simulink model "rx_channelizer_AIE"  (R2024a)
settings: Solver=VariableStepAuto  StartTime=0.0  StopTime=1280*12/fs  RelTol=1e-3
PreLoadFcn:
  | ch_rate = 41e6; % per channel sample rate
  | num_ch = 32;
  | 
  | % note:  6 coeffs/ch;
  | fs = ch_rate*num_ch;
  | sample_rate = 1/fs;
  | base_freq=1e6; % what base channel frequency to modulate?
  | 
  | generate_prototype_FIR; % create FIR coeffs
values from neighbouring files (symbols this model uses):
  ch0f = int16(scale*ch0)    [generate_prototype_FIR.m]
  ch10f = int16(scale*ch10)    [generate_prototype_FIR.m]
  ch11f = int16(scale*ch11)    [generate_prototype_FIR.m]
  ch12f = int16(scale*ch12)    [generate_prototype_FIR.m]
  ch13f = int16(scale*ch13)    [generate_prototype_FIR.m]
  ch14f = int16(scale*ch14)    [generate_prototype_FIR.m]
  ch15f = int16(scale*ch15)    [generate_prototype_FIR.m]
  ch16f = int16(scale*ch16)    [generate_prototype_FIR.m]
  ch17f = int16(scale*ch17)    [generate_prototype_FIR.m]
  ch18f = int16(scale*ch18)    [generate_prototype_FIR.m]
  ch19f = int16(scale*ch19)    [generate_prototype_FIR.m]
  ch1f = int16(scale*ch1)    [generate_prototype_FIR.m]
  ch20f = int16(scale*ch20)    [generate_prototype_FIR.m]
  ch21f = int16(scale*ch21)    [generate_prototype_FIR.m]
  ch22f = int16(scale*ch22)    [generate_prototype_FIR.m]
  ch23f = int16(scale*ch23)    [generate_prototype_FIR.m]
  ch24f = int16(scale*ch24)    [generate_prototype_FIR.m]
  ch25f = int16(scale*ch25)    [generate_prototype_FIR.m]
  ch26f = int16(scale*ch26)    [generate_prototype_FIR.m]
  ch27f = int16(scale*ch27)    [generate_prototype_FIR.m]
  ch28f = int16(scale*ch28)    [generate_prototype_FIR.m]
  ch29f = int16(scale*ch29)    [generate_prototype_FIR.m]
  ch2f = int16(scale*ch2)    [generate_prototype_FIR.m]
  ch30f = int16(scale*ch30)    [generate_prototype_FIR.m]
  ch31f = int16(scale*ch31)    [generate_prototype_FIR.m]
  ch3f = int16(scale*ch3)    [generate_prototype_FIR.m]
  ch4f = int16(scale*ch4)    [generate_prototype_FIR.m]
  ch5f = int16(scale*ch5)    [generate_prototype_FIR.m]
  ch6f = int16(scale*ch6)    [generate_prototype_FIR.m]
  ch7f = int16(scale*ch7)    [generate_prototype_FIR.m]
  ch8f = int16(scale*ch8)    [generate_prototype_FIR.m]
  ch9f = int16(scale*ch9)    [generate_prototype_FIR.m]
  filtAIE1_fp = filtAIE2_fp'    [generate_prototype_FIR.m]
undefined symbols (not defined in the file or in its folder): None, PLclk, S, vsva2197, xcvc1902
libraries: aieBasic x12, dspsrcs4 x4, aieUtilities x4, aieDSP x2, dspmlti4 x1, dspxfrm3 x1, vmcUtilities x1
settings Model: Creator=mmi  LastModifiedBy=robg
settings SolverCC: AlgebraicLoopSolver=TrustRegion
settings DebuggingCC: UnconnectedInputMsg=warning  UnconnectedOutputMsg=warning  UnconnectedLineMsg=warning
settings HardwareCC: ProdBitPerPointer=32  ProdBitPerSizeT=32  ProdBitPerPtrDiffT=32  ProdLargestAtomicFloat=None  ProdIntDivRoundTo=Undefined  ProdEndianess=Unspecified  ProdWordSize=32  ProdHWDeviceType=ASIC/FPGA->ASIC/FPGA  TargetBitPerLong=64  TargetBitPerPointer=64  TargetBitPerSizeT=64  TargetBitPerPtrDiffT=64  TargetLongLongMode=on  TargetIntDivRoundTo=Zero  TargetEndianess=LittleEndian  TargetWordSize=64  TargetHWDeviceType=Custom Processor->MATLAB Host Computer  ProdEqTarget=off
settings ModelReferenceCC: EnableRefExpFcnMdlSchedulingChecks=on
settings RTWCC: GPUComputeCapability=3.5  DLArmComputeVersion=19.05
settings ConfigComp: CovBoundaryAbsTol=1.0e-5

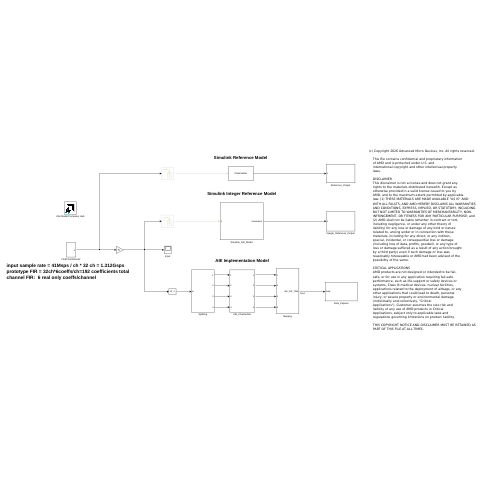
[thumbnail: Simulink's stored preview of the top-level diagram]
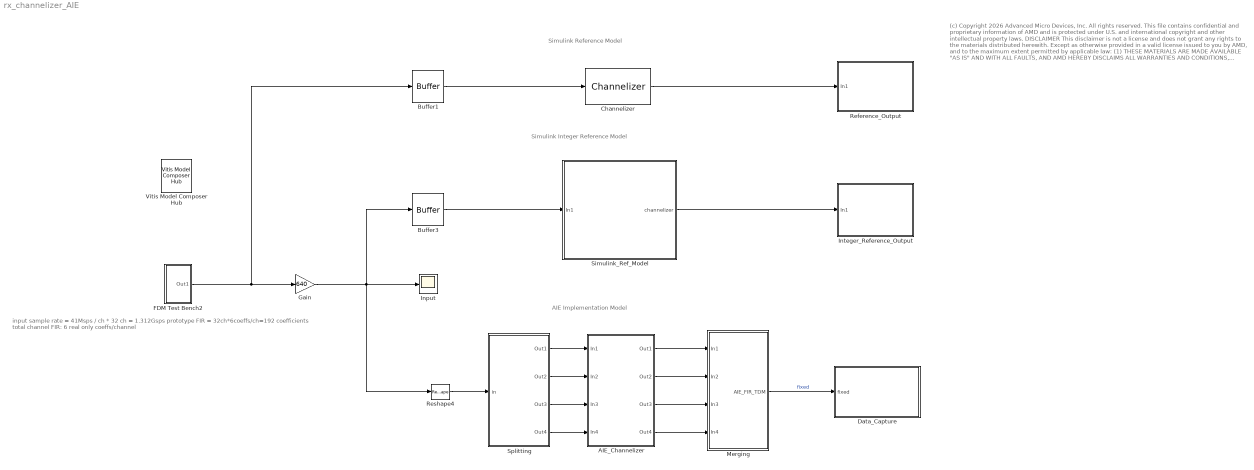
== system rx_channelizer_AIE ==
  note: input sample rate = 41Msps / ch * 32 ch = 1.312Gsps
      | prototype FIR = 32ch*6coeffs/ch=192 coefficients total
      | channel FIR: 6 real only coeffs/channel
  note: (c) Copyright 2026 Advanced Micro Devices, Inc. All rights reserved.
      |
      | This file contains confidential and proprietary information
      | of AMD and is protected under U.S. and
      | international copyright and other intellectual property
      | laws.
      |
      | DISCLAIMER
      | This disclaimer is not a license and does not grant any
      | rights to the materials distributed herewith. Except as
      | otherwise provided in a valid license issued to you by
      | AMD, and to the maximum extent permitted by applicable
      | law: (1) THESE MATERIALS ARE MADE AVAILABLE "AS IS" AND
      | WITH ALL FAULTS, AND AMD HEREBY DISCLAIMS ALL WARRANTIES
      | AND CONDITIONS, EXPRESS, IMPLIED, OR STATUTORY, INCLUDING
      | BUT NOT LIMITED TO WARRANTIES OF MERCHANTABILITY, NON-
      | INFRINGEMENT, OR FITNESS FOR ANY PARTICULAR PURPOSE; and
      | (2) AMD shall not be liable (whether in contract or tort,
      | including negligence, or under any other theory of
      | liability) for any loss or damage of any kind or nature
      | related to, arising under or in connection with these
      | materials, including for any direct, or any indirect,
      | special, incidental, or consequential loss or damage
      | (including loss of data, profits, goodwill, or any type of
      | loss or damage suffered as a result of any action brought
      | by a third party) even if such damage or loss was
      | reasonably foreseeable or AMD had been advised of the
      | possibility of the same.
      |
      | CRITICAL APPLICATIONS
      | AMD products are not designed or intended to be fail-
      | safe, or for use in any application requiring fail-safe
      | performance, such as life-support or safety devices or
      | systems, Class III medical devices, nuclear facilities,
      | applications related to the deployment of airbags, or any
      | other applications that could lead to death, personal
      | injury, or severe property or environmental damage
      | (individually and collectively, "Critical
      | Applications"). Customer assumes the sole risk and
      | liability of any use of AMD products in Critical
      | Applications, subject only to applicable laws and
      | regulations governing limitations on product liability.
      |
      | THIS COPYRIGHT NOTICE AND DISCLAIMER MUST BE RETAINED AS
      | PART OF THIS FILE AT ALL TIMES.
  note: Simulink Reference Model
  note: Simulink Integer Reference Model
  note: AIE Implementation Model
  AIE_Channelizer : Subsystem
  Buffer1 : Buffer  N=num_ch  OutputFrames=off
  Buffer3 : Buffer  N=num_ch  OutputFrames=off
  Channelizer : dspmlti4/Channelizer  NumFrequencyBands=32  DecimationFactor=Number of frequency bands  Specification=Coefficients  CoefficientsPort=off  NumTapsPerBand=6  StopbandAttenuation=80  LowpassCoefficients=pf  AllowArbitraryInputLength=off  BandsAsSeparateOutputPorts=off  SimulateUsing=Interpreted execution
  Data_Capture : Subsystem
  FDM Test Bench2 : Subsystem
  Gain : Gain  Gain=640  OutDataTypeStr=int16
  Input : Scope
  Integer_Reference_Output : Subsystem
  Merging : Subsystem
  Reference_Output : Subsystem
  Reshape4 : Reshape
  Simulink_Ref_Model : Subsystem
  Splitting : Subsystem
  Vitis Model Composer Hub : vmcUtilities/Vitis Model Composer Hub  Tag=genX  CodeGeneration=off  SubsystemName=AIEchannelizer  BlockHierPath=rx_channelizer_AIE/AIEchannelizer  CompilationType=HDLCompilation  SubsystemType=AIENode  ExportTypeV2=IP Catalog  StartColumn=1  NumberOfColumns=1  TargetDirectory=./code_AIE_rr  exportDesign=off  analyzeDesign=on  validateDesignOnHw=off  ExportType=AI Engines  IpVendor=xilinx.com  IpLibrary=hls  IpVersion=1.0  IpHWLanguage=Verilog  AieCompilerOptions={}  AieSimulatorOptions={}  CreateTestbench=on  TestbenchStackSize=10  RunRtlSim=off  RunCSim=off  RunAieSim=off  AieSimTimeout=50000  RunAieSimProfiling=off  LaunchVitisAnalyzer=off  PlotOutput=off  RunX86Sim=off  X86SimTimeout=10  GenHwImage=off  GenLibadfXo=off  GenHwValidationCode=off  PlatformType=Not Specified  HwSystemType=Baremetal  HwValidationTarget=hw  ProjDevice=Versal VCK190 Evaluation Platform with New SD Level Shifter (xcvc1902-vsva2197-2MP-e-S)  ProjDevicePart=xcvc1902-vsva2197-2MP-e-S  AIEType=AIE  SamplePeriod=-1  ClockFrequency=200  DataPathParallelism=1  xilinxfamily=versalaicore  part=xcvc1902  speed=-2MP-e-S  package=vsva2197  directory=./netlist/ip/PL_Channelizer/src  testbench=off  incr_netlist=off  synthesis_tool=Vivado  clock_wrapper=Clock Enables  dbl_ovrd=According to Block Masks  dcm_input_clock_period=10  sysclk_period=1e9/PLclk  simulink_period=1/(ch_rate*16)  eval_field=0  IPInfoJsonString="{\"DUTSubsystemName\":\"AIEchannelizer\",\"AIESubsystem\":{\"SubsystemName\":\"AIEchannelizer\",\"TargetDirectory\":\"./code_AIE_rr\",\"AIEArrayConfig\":\"Use entire AIE array\",\"StartColumn\":\"0\",\"NumberOfColumns\":\"1\"},\"SubsystemTag\":\"AIENode\"}"  LogFileName=/home/mmi/xmc/basics/Channelizer/WTS/code_AIE_rr/model_composer.log  NThreads=4  IPConfigFile=/tmp/vmctmp-7854972894121886229/rx_channelizer_AIE_ipconfig.json
  wires:
  Buffer1/1 -> Channelizer/1
  Buffer3/1 -> Simulink_Ref_Model/1(In1)
  Reshape4/1 -> Splitting/1(in)
  AIE_Channelizer/4(Out4) -> Merging/4(In4)
  Splitting/4(Out4) -> AIE_Channelizer/4(In4)
  Gain/1 -> Buffer3/1, Input/1, Reshape4/1
  AIE_Channelizer/2(Out2) -> Merging/2(In2)
  Splitting/2(Out2) -> AIE_Channelizer/2(In2)
  Splitting/3(Out3) -> AIE_Channelizer/3(In3)
  AIE_Channelizer/3(Out3) -> Merging/3(In3)
  Splitting/1(Out1) -> AIE_Channelizer/1(In1)
  AIE_Channelizer/1(Out1) -> Merging/1(In1)
  FDM Test Bench2/1(Out1) -> Buffer1/1, Gain/1
  Merging/1(AIE_FIR_TDM) -> Data_Capture/1(fixed)  "fixed"
  Simulink_Ref_Model/1(channelizer) -> Integer_Reference_Output/1(In1)
  Channelizer/1 -> Reference_Output/1(In1)

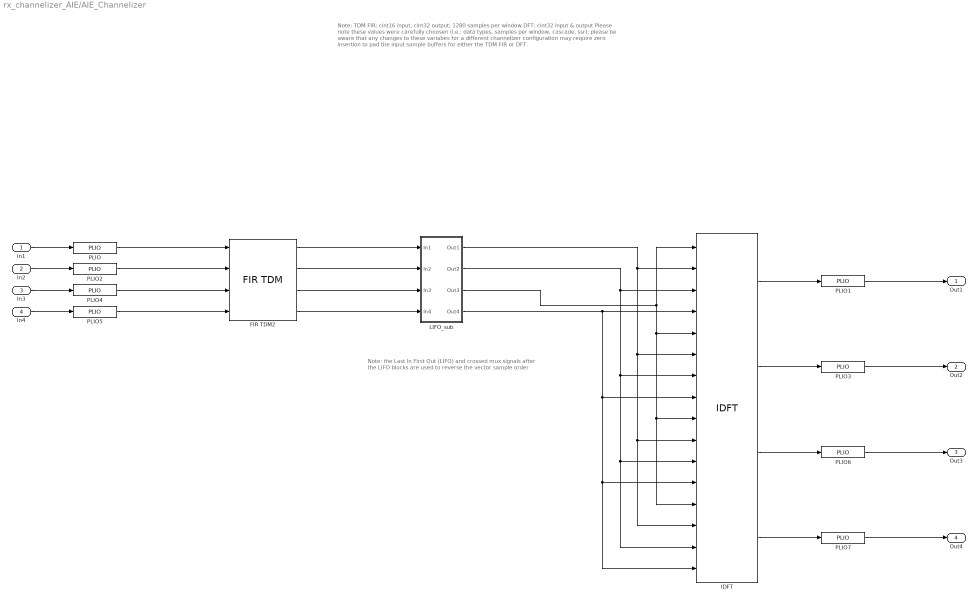
== system rx_channelizer_AIE/AIE_Channelizer ==
  note: Note: the Last In First Out (LIFO) and crossed mux signals after the LIFO blocks are used to reverse the vector sample order
  note: Note:
      | TDM FIR: cint16 input, cint32 output; 1280 samples per window
      | DFT: cint32 input & output
      |
      | Please note these values were carefully choosen (i.e.: data types, samples per window, cascade, ssr); please be aware that any changes to these variabes for a different channelizer configuration may require zero insertion to pad the input sample buffers for either the TDM FIR or DFT.
  In1 : Inport
  In2 : Inport  Port=2
  In3 : Inport  Port=3
  In4 : Inport  Port=4
  FIR TDM2 : aieDSP/FIR TDM  data_type=cint16  data_out_type=cint32  coef_type=int16  use_coeff_reload=off  fir_length=6  coeff=[filtAIE1_fp]  shift_val=0  rnd_mode=Floor  input_window_size=1280  tdm_channels=32  sat_mode=0-None  casc_length=1  ssr=4  AIE_VARIANT=1  TP_API=0  dual_ip=0  TP_NUM_OUTPUTS=0  blockJsonConstraints=[]  blockJsonConstraintsInternal=[]  spec=vmc_fir_tdm.json  SerializedMaskParamNames=[]  SerializedMaskParamValues=[]  SerializedMaskParamVisibilities=[]  block_type=FIR TDM  SerializedMaskParamDataypes=typename|typename|typename|uint|uint|coef_type|uint|uint|uint|uint|uint|uint|uint|uint|uint|uint|uint  SerializedMaskParamEnumStrArr=0|0|0|0|0|0|0|Floor,Ceiling,Round to positive infinity,Round to negative infinity,Round symmetrical to infinity,Round symmetrical to zero,Round convergent to even,Round convergent to odd|0|0|0-None,1-Asymmetric,3-Symmetric|0|0|0|0|0|0  SerializedMaskParamEnumValArr=0|0|0|0|0|0|0|0,1,2,3,4,5,6,7|0|0|0,1,3|0|0|0|0|0|0  SerializedMaskParamVectorArr=0|0|0|0|0|1|0|0|0|0|0|0|0|0|0|0|0  SerializedMaskParamKeys=TT_DATA|TT_OUT_DATA|TT_COEFF|TP_USE_COEFF_RELOAD|TP_FIR_LEN|coeff|TP_SHIFT|TP_RND|TP_INPUT_WINDOW_VSIZE|TP_TDM_CHANNELS|TP_SAT|TP_CASC_LEN|TP_SSR|AIE_VARIANT|TP_API|TP_DUAL_IP|TP_NUM_OUTPUTS
  IDFT : aieDSP/IDFT  data_type=cint32  twiddle_type=cint16  point_size=32  num_frames=40  shift_val=5  rnd_mode=Floor  ssr=4  sat_mode=0-None  casc_length=4  AIE_VARIANT=1  TP_API=0  TP_FFT_NIFFT=0  blockJsonConstraints=[]  blockJsonConstraintsInternal=[]  spec=vmc_idft.json  SerializedMaskParamNames=[]  SerializedMaskParamValues=[]  SerializedMaskParamVisibilities=[]  block_type=IDFT  SerializedMaskParamDataypes=typename|typename|uint|uint|uint|uint|uint|uint|uint|uint|uint|uint  SerializedMaskParamEnumStrArr=0|0|0|0|0|Floor,Ceiling,Round to positive infinity,Round to negative infinity,Round symmetrical to infinity,Round symmetrical to zero,Round convergent to even,Round convergent to odd|0|0-None,1-Asymmetric,3-Symmetric|0|0|0|0  SerializedMaskParamEnumValArr=0|0|0|0|0|0,1,2,3,4,5,6,7|0|0,1,3|0|0|0|0  SerializedMaskParamVectorArr=0|0|0|0|0|0|0|0|0|0|0|0  SerializedMaskParamKeys=TT_DATA|TT_TWIDDLE|TP_POINT_SIZE|TP_NUM_FRAMES|TP_SHIFT|TP_RND|TP_SSR|TP_SAT|TP_CASC_LEN|AIE_VARIANT|TP_API|TP_FFT_NIFFT
  LIFO_sub : Subsystem
  PLIO{,1..7} (8 alike) : aieBasic/PLIO  PlioWidth=64  PlioFreqSpec=on  PlioFreq=625  ColLocation=0  channel=0  blockJsonConstraints=[]  deprecateConstraints=0
  Out1 : Outport
  Out2 : Outport  Port=2
  Out3 : Outport  Port=3
  Out4 : Outport  Port=4
  wires:
  PLIO1/1 -> Out1/1
  In1/1 -> PLIO/1
  In2/1 -> PLIO2/1
  PLIO3/1 -> Out2/1
  In3/1 -> PLIO4/1
  In4/1 -> PLIO5/1
  IDFT/1 -> PLIO1/1
  IDFT/2 -> PLIO3/1
  PLIO/1 -> FIR TDM2/1
  PLIO2/1 -> FIR TDM2/2
  PLIO4/1 -> FIR TDM2/3
  PLIO5/1 -> FIR TDM2/4
  PLIO6/1 -> Out3/1
  IDFT/4 -> PLIO7/1
  IDFT/3 -> PLIO6/1
  PLIO7/1 -> Out4/1
  LIFO_sub/4(Out4) -> IDFT/8, IDFT/16, IDFT/12, IDFT/4
  LIFO_sub/2(Out2) -> IDFT/3, IDFT/7, IDFT/11, IDFT/15
  LIFO_sub/1(Out1) -> IDFT/6, IDFT/14, IDFT/10, IDFT/2
  LIFO_sub/3(Out3) -> IDFT/1, IDFT/5, IDFT/9, IDFT/13
  FIR TDM2/1 -> LIFO_sub/1(In1)
  FIR TDM2/2 -> LIFO_sub/2(In2)
  FIR TDM2/3 -> LIFO_sub/3(In3)
  FIR TDM2/4 -> LIFO_sub/4(In4)

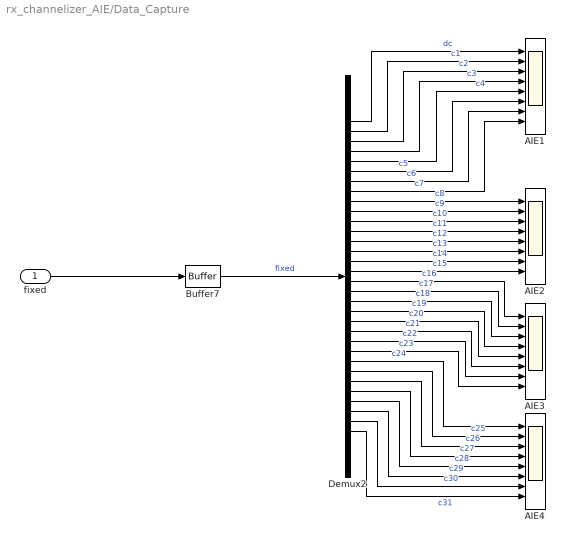
== system rx_channelizer_AIE/Data_Capture ==
  fixed : Inport
  AIE{1..4} (4 alike) : Scope  NumInputPorts=8
  Buffer7 : Buffer  N=32  OutputFrames=off
  Demux2 : Demux  Outputs=num_ch
  wires:
  Demux2/23 -> AIE3/7  "c22"
  Demux2/1 -> AIE1/1  "dc"
  Demux2/28 -> AIE4/4  "c27"
  Demux2/13 -> AIE2/5  "c12"
  fixed/1 -> Buffer7/1
  Demux2/29 -> AIE4/5  "c28"
  Demux2/24 -> AIE3/8  "c23"
  Demux2/25 -> AIE4/1  "c24"
  Demux2/2 -> AIE1/2  "c1"
  Demux2/14 -> AIE2/6  "c13"
  Demux2/7 -> AIE1/7  "c6"
  Demux2/27 -> AIE4/3  "c26"
  Demux2/20 -> AIE3/4  "c19"
  Demux2/30 -> AIE4/6  "c29"
  Buffer7/1 -> Demux2/1  "fixed"
  Demux2/32 -> AIE4/8  "c31"
  Demux2/22 -> AIE3/6  "c21"
  Demux2/31 -> AIE4/7  "c30"
  Demux2/10 -> AIE2/2  "c9"
  Demux2/12 -> AIE2/4  "c11"
  Demux2/4 -> AIE1/4  "c3"
  Demux2/15 -> AIE2/7  "c14"
  Demux2/19 -> AIE3/3  "c18"
  Demux2/6 -> AIE1/6  "c5"
  Demux2/8 -> AIE1/8  "c7"
  Demux2/5 -> AIE1/5  "c4"
  Demux2/26 -> AIE4/2  "c25"
  Demux2/9 -> AIE2/1  "c8"
  Demux2/11 -> AIE2/3  "c10"
  Demux2/16 -> AIE2/8  "c15"
  Demux2/3 -> AIE1/3  "c2"
  Demux2/21 -> AIE3/5  "c20"
  Demux2/17 -> AIE3/1  "c16"
  Demux2/18 -> AIE3/2  "c17"

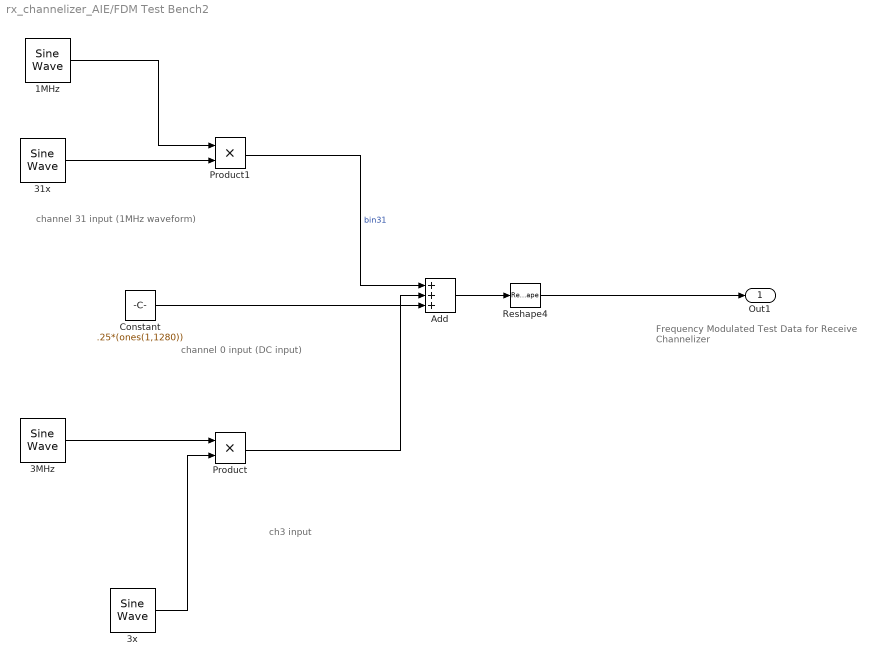
== system rx_channelizer_AIE/FDM Test Bench2 ==
  note: ch3 input
  note: Frequency Modulated Test Data for Receive Channelizer
  note: channel 0 input (DC input)
  note: channel 31 input (1MHz waveform)
  1MHz : dspsrcs4/Sine Wave  Amplitude=0.5  Frequency=base_freq  Phase=0  SampleMode=Discrete  OutComplex=Complex  CompMethod=Trigonometric fcn  TableSize=Speed  SampleTime=1/fs  SamplesPerFrame=1280  ResetState=Restart at time zero  OutputFrames=off  dataType=double  wordLen=16  udDataType=sfix(16)  fracBitsMode=Best precision  numFracBits=15  OutDataTypeStr=double  LastOutDataTypeStr=double
  31x : dspsrcs4/Sine Wave  Amplitude=0.25  Frequency=31*ch_rate  Phase=0  SampleMode=Discrete  OutComplex=Complex  CompMethod=Trigonometric fcn  TableSize=Speed  SampleTime=1/fs  SamplesPerFrame=1280  ResetState=Restart at time zero  OutputFrames=off  dataType=double  wordLen=16  udDataType=sfix(16)  fracBitsMode=Best precision  numFracBits=15  OutDataTypeStr=double  LastOutDataTypeStr=double
  3MHz : dspsrcs4/Sine Wave  Amplitude=0.5  Frequency=base_freq*3  Phase=0  SampleMode=Discrete  OutComplex=Complex  CompMethod=Trigonometric fcn  TableSize=Speed  SampleTime=1/fs  SamplesPerFrame=1280  ResetState=Restart at time zero  OutputFrames=off  dataType=double  wordLen=16  udDataType=sfix(16)  fracBitsMode=Best precision  numFracBits=15  OutDataTypeStr=double  LastOutDataTypeStr=double
  3x : dspsrcs4/Sine Wave  Amplitude=0.5  Frequency=3*ch_rate  Phase=0  SampleMode=Discrete  OutComplex=Complex  CompMethod=Trigonometric fcn  TableSize=Speed  SampleTime=1/fs  SamplesPerFrame=1280  ResetState=Restart at time zero  OutputFrames=off  dataType=double  wordLen=16  udDataType=sfix(16)  fracBitsMode=Best precision  numFracBits=15  OutDataTypeStr=double  LastOutDataTypeStr=double
  Add : Sum  Inputs=+++
  Constant : Constant  Value=.25*(ones(1,1280))  SampleTime=1280/fs
  Product : Product
  Product1 : Product
  Reshape4 : Reshape
  Out1 : Outport
  wires:
  3x/1 -> Product/2
  1MHz/1 -> Product1/1
  Product1/1 -> Add/1  "bin31"
  Product/1 -> Add/2
  31x/1 -> Product1/2
  Add/1 -> Reshape4/1
  3MHz/1 -> Product/1
  Constant/1 -> Add/3
  Reshape4/1 -> Out1/1

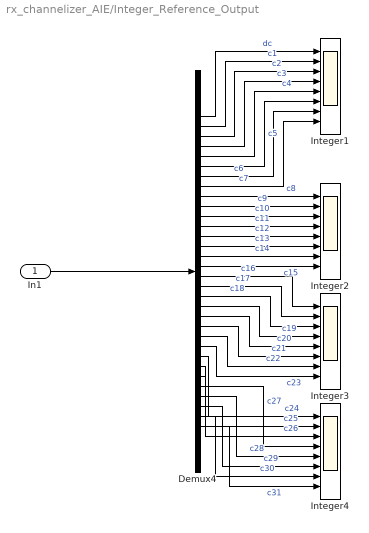
== system rx_channelizer_AIE/Integer_Reference_Output ==
  In1 : Inport
  Demux4 : Demux  Outputs=num_ch
  Integer{1..4} (4 alike) : Scope  NumInputPorts=8
  wires:
  Demux4/23 -> Integer3/7  "c22"
  Demux4/4 -> Integer1/4  "c3"
  Demux4/7 -> Integer1/7  "c6"
  Demux4/29 -> Integer4/5  "c28"
  Demux4/14 -> Integer2/6  "c13"
  Demux4/20 -> Integer3/4  "c19"
  Demux4/8 -> Integer1/8  "c7"
  Demux4/11 -> Integer2/3  "c10"
  Demux4/5 -> Integer1/5  "c4"
  Demux4/10 -> Integer2/2  "c9"
  Demux4/9 -> Integer2/1  "c8"
  Demux4/32 -> Integer4/8  "c31"
  Demux4/24 -> Integer3/8  "c23"
  Demux4/28 -> Integer4/4  "c27"
  Demux4/15 -> Integer2/7  "c14"
  Demux4/16 -> Integer2/8  "c15"
  In1/1 -> Demux4/1
  Demux4/12 -> Integer2/4  "c11"
  Demux4/27 -> Integer4/3  "c26"
  Demux4/13 -> Integer2/5  "c12"
  Demux4/6 -> Integer1/6  "c5"
  Demux4/30 -> Integer4/6  "c29"
  Demux4/21 -> Integer3/5  "c20"
  Demux4/31 -> Integer4/7  "c30"
  Demux4/3 -> Integer1/3  "c2"
  Demux4/26 -> Integer4/2  "c25"
  Demux4/22 -> Integer3/6  "c21"
  Demux4/2 -> Integer1/2  "c1"
  Demux4/19 -> Integer3/3  "c18"
  Demux4/25 -> Integer4/1  "c24"
  Demux4/17 -> Integer3/1  "c16"
  Demux4/18 -> Integer3/2  "c17"
  Demux4/1 -> Integer1/1  "dc"

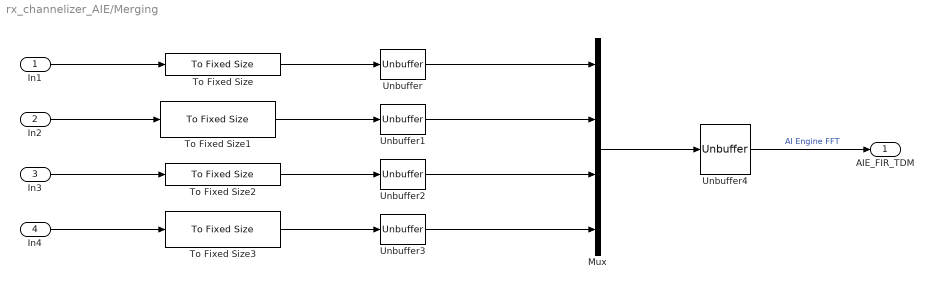
== system rx_channelizer_AIE/Merging ==
  In1 : Inport
  In2 : Inport  Port=2
  In3 : Inport  Port=3
  In4 : Inport  Port=4
  Mux : Mux
  To Fixed Size{,1..3} (4 alike) : aieUtilities/To Fixed Size  Mode=Stop simulation when input variable-size signal is not full  OutputSize=Inherit: Same as input  CopyMethod=Buffer samples to form output  HasStatusOutput=on
  Unbuffer{,1..4} (5 alike) : Unbuffer
  AIE_FIR_TDM : Outport
  wires:
  To Fixed Size1/1 -> Unbuffer1/1
  In2/1 -> To Fixed Size1/1
  To Fixed Size/1 -> Unbuffer/1
  Mux/1 -> Unbuffer4/1
  Unbuffer4/1 -> AIE_FIR_TDM/1  "AI Engine FFT"
  In1/1 -> To Fixed Size/1
  To Fixed Size2/1 -> Unbuffer2/1
  In3/1 -> To Fixed Size2/1
  In4/1 -> To Fixed Size3/1
  To Fixed Size3/1 -> Unbuffer3/1
  Unbuffer/1 -> Mux/1
  Unbuffer1/1 -> Mux/2
  Unbuffer2/1 -> Mux/3
  Unbuffer3/1 -> Mux/4

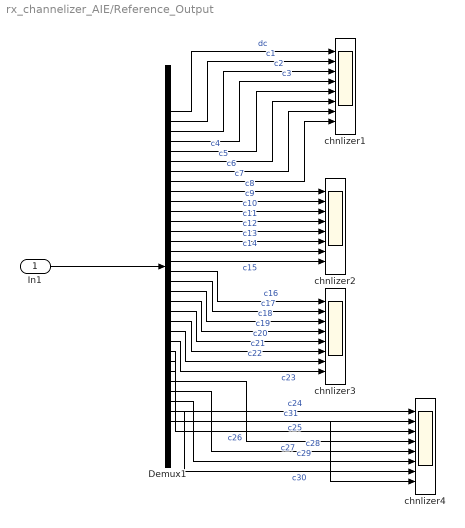
== system rx_channelizer_AIE/Reference_Output ==
  In1 : Inport
  Demux1 : Demux  Outputs=num_ch
  chnlizer{1..4} (4 alike) : Scope  NumInputPorts=8
  wires:
  Demux1/32 -> chnlizer4/8  "c31"
  Demux1/22 -> chnlizer3/6  "c21"
  Demux1/8 -> chnlizer1/8  "c7"
  Demux1/25 -> chnlizer4/1  "c24"
  Demux1/15 -> chnlizer2/7  "c14"
  Demux1/17 -> chnlizer3/1  "c16"
  Demux1/26 -> chnlizer4/2  "c25"
  Demux1/20 -> chnlizer3/4  "c19"
  Demux1/14 -> chnlizer2/6  "c13"
  Demux1/6 -> chnlizer1/6  "c5"
  Demux1/1 -> chnlizer1/1  "dc"
  Demux1/31 -> chnlizer4/7  "c30"
  Demux1/10 -> chnlizer2/2  "c9"
  Demux1/24 -> chnlizer3/8  "c23"
  Demux1/18 -> chnlizer3/2  "c17"
  Demux1/4 -> chnlizer1/4  "c3"
  In1/1 -> Demux1/1
  Demux1/19 -> chnlizer3/3  "c18"
  Demux1/27 -> chnlizer4/3  "c26"
  Demux1/11 -> chnlizer2/3  "c10"
  Demux1/16 -> chnlizer2/8  "c15"
  Demux1/23 -> chnlizer3/7  "c22"
  Demux1/30 -> chnlizer4/6  "c29"
  Demux1/21 -> chnlizer3/5  "c20"
  Demux1/9 -> chnlizer2/1  "c8"
  Demux1/13 -> chnlizer2/5  "c12"
  Demux1/29 -> chnlizer4/5  "c28"
  Demux1/12 -> chnlizer2/4  "c11"
  Demux1/28 -> chnlizer4/4  "c27"
  Demux1/5 -> chnlizer1/5  "c4"
  Demux1/7 -> chnlizer1/7  "c6"
  Demux1/3 -> chnlizer1/3  "c2"
  Demux1/2 -> chnlizer1/2  "c1"

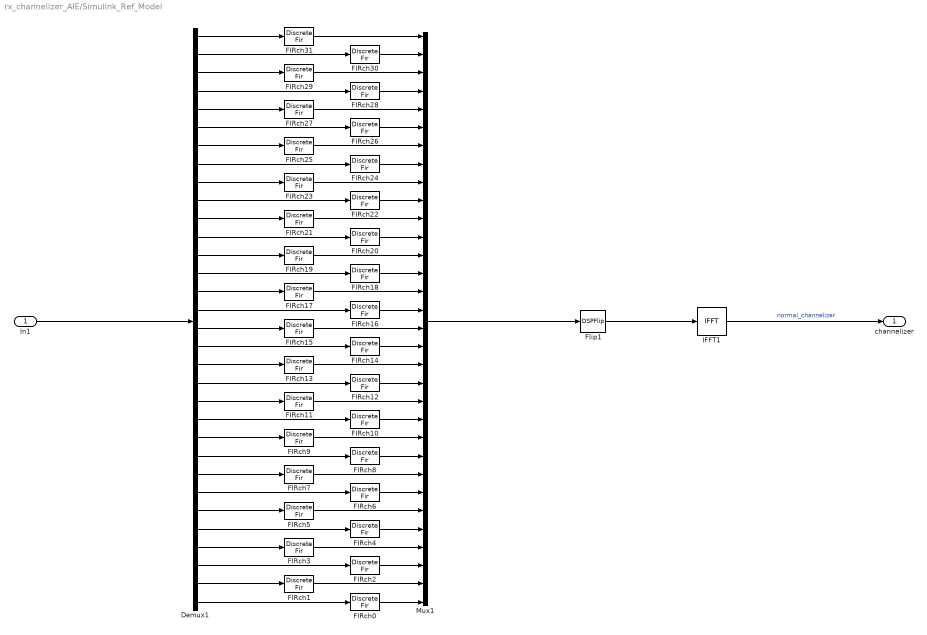
== system rx_channelizer_AIE/Simulink_Ref_Model ==
  In1 : Inport
  Demux1 : Demux  Outputs=num_ch
  FIRch0 : DiscreteFir  Coefficients=[ch0f]  InputProcessing=Columns as channels (frame based)  CoefDataTypeStr=int16  OutDataTypeStr=int32
  FIRch1 : DiscreteFir  Coefficients=[ch1f]  InputProcessing=Columns as channels (frame based)  CoefDataTypeStr=int16  OutDataTypeStr=int32
  FIRch10 : DiscreteFir  Coefficients=[ch10f]  InputProcessing=Columns as channels (frame based)  CoefDataTypeStr=int16  OutDataTypeStr=int32
  FIRch11 : DiscreteFir  Coefficients=[ch11f]  InputProcessing=Columns as channels (frame based)  CoefDataTypeStr=int16  OutDataTypeStr=int32
  FIRch12 : DiscreteFir  Coefficients=[ch12f]  InputProcessing=Columns as channels (frame based)  CoefDataTypeStr=int16  OutDataTypeStr=int32
  FIRch13 : DiscreteFir  Coefficients=[ch13f]  InputProcessing=Columns as channels (frame based)  CoefDataTypeStr=int16  OutDataTypeStr=int32
  FIRch14 : DiscreteFir  Coefficients=[ch14f]  InputProcessing=Columns as channels (frame based)  CoefDataTypeStr=int16  OutDataTypeStr=int32
  FIRch15 : DiscreteFir  Coefficients=[ch15f]  InputProcessing=Columns as channels (frame based)  CoefDataTypeStr=int16  OutDataTypeStr=int32
  FIRch16 : DiscreteFir  Coefficients=[ch16f]  InputProcessing=Columns as channels (frame based)  CoefDataTypeStr=int16  OutDataTypeStr=int32
  FIRch17 : DiscreteFir  Coefficients=[ch17f]  InputProcessing=Columns as channels (frame based)  CoefDataTypeStr=int16  OutDataTypeStr=int32
  FIRch18 : DiscreteFir  Coefficients=[ch18f]  InputProcessing=Columns as channels (frame based)  CoefDataTypeStr=int16  OutDataTypeStr=int32
  FIRch19 : DiscreteFir  Coefficients=[ch19f]  InputProcessing=Columns as channels (frame based)  CoefDataTypeStr=int16  OutDataTypeStr=int32
  FIRch2 : DiscreteFir  Coefficients=[ch2f]  InputProcessing=Columns as channels (frame based)  CoefDataTypeStr=int16  OutDataTypeStr=int32
  FIRch20 : DiscreteFir  Coefficients=[ch20f]  InputProcessing=Columns as channels (frame based)  CoefDataTypeStr=int16  OutDataTypeStr=int32
  FIRch21 : DiscreteFir  Coefficients=[ch21f]  InputProcessing=Columns as channels (frame based)  CoefDataTypeStr=int16  OutDataTypeStr=int32
  FIRch22 : DiscreteFir  Coefficients=[ch22f]  InputProcessing=Columns as channels (frame based)  CoefDataTypeStr=int16  OutDataTypeStr=int32
  FIRch23 : DiscreteFir  Coefficients=[ch23f]  InputProcessing=Columns as channels (frame based)  CoefDataTypeStr=int16  OutDataTypeStr=int32
  FIRch24 : DiscreteFir  Coefficients=[ch24f]  InputProcessing=Columns as channels (frame based)  CoefDataTypeStr=int16  OutDataTypeStr=int32
  FIRch25 : DiscreteFir  Coefficients=[ch25f]  InputProcessing=Columns as channels (frame based)  CoefDataTypeStr=int16  OutDataTypeStr=int32
  FIRch26 : DiscreteFir  Coefficients=[ch26f]  InputProcessing=Columns as channels (frame based)  CoefDataTypeStr=int16  OutDataTypeStr=int32
  FIRch27 : DiscreteFir  Coefficients=[ch27f]  InputProcessing=Columns as channels (frame based)  CoefDataTypeStr=int16  OutDataTypeStr=int32
  FIRch28 : DiscreteFir  Coefficients=[ch28f]  InputProcessing=Columns as channels (frame based)  CoefDataTypeStr=int16  OutDataTypeStr=int32
  FIRch29 : DiscreteFir  Coefficients=[ch29f]  InputProcessing=Columns as channels (frame based)  CoefDataTypeStr=int16  OutDataTypeStr=int32
  FIRch3 : DiscreteFir  Coefficients=[ch3f]  InputProcessing=Columns as channels (frame based)  CoefDataTypeStr=int16  OutDataTypeStr=int32
  FIRch30 : DiscreteFir  Coefficients=[ch30f]  InputProcessing=Columns as channels (frame based)  CoefDataTypeStr=int16  OutDataTypeStr=int32
  FIRch31 : DiscreteFir  Coefficients=[ch31f]  InputProcessing=Columns as channels (frame based)  CoefDataTypeStr=int16  OutDataTypeStr=int32
  FIRch4 : DiscreteFir  Coefficients=[ch4f]  InputProcessing=Columns as channels (frame based)  CoefDataTypeStr=int16  OutDataTypeStr=int32
  FIRch5 : DiscreteFir  Coefficients=[ch5f]  InputProcessing=Columns as channels (frame based)  CoefDataTypeStr=int16  OutDataTypeStr=int32
  FIRch6 : DiscreteFir  Coefficients=[ch6f]  InputProcessing=Columns as channels (frame based)  CoefDataTypeStr=int16  OutDataTypeStr=int32
  FIRch7 : DiscreteFir  Coefficients=[ch7f]  InputProcessing=Columns as channels (frame based)  CoefDataTypeStr=int16  OutDataTypeStr=int32
  FIRch8 : DiscreteFir  Coefficients=[ch8f]  InputProcessing=Columns as channels (frame based)  CoefDataTypeStr=int16  OutDataTypeStr=int32
  FIRch9 : DiscreteFir  Coefficients=[ch9f]  InputProcessing=Columns as channels (frame based)  CoefDataTypeStr=int16  OutDataTypeStr=int32
  Flip1 : DSPFlip
  IFFT1 : dspxfrm3/IFFT  FFTImplementation=Auto  CompMethod=Table lookup  TableOpt=NEW  TableOptActive=Speed  BitRevOrder=off  cs_in=off  Normalize=off  InheritFFTLength=on  FFTLength=64  WrapInput=on  mode=Real  outSamplingMode=Sample based  roundingMode=Ceiling  overflowMode=off  firstCoeffDataTypeStr=Inherit: Same word length as input  firstCoeffLastDataTypeStr=Inherit: Same word length as input  outputMin=[]  outputMax=[]
  Mux1 : Mux  Inputs=num_ch
  channelizer : Outport
  wires:
  In1/1 -> Demux1/1
  Demux1/1 -> FIRch31/1
  FIRch31/1 -> Mux1/1
  Demux1/2 -> FIRch30/1
  FIRch30/1 -> Mux1/2
  Demux1/3 -> FIRch29/1
  FIRch29/1 -> Mux1/3
  Demux1/4 -> FIRch28/1
  FIRch28/1 -> Mux1/4
  Demux1/5 -> FIRch27/1
  FIRch27/1 -> Mux1/5
  FIRch26/1 -> Mux1/6
  Demux1/6 -> FIRch26/1
  Demux1/7 -> FIRch25/1
  FIRch25/1 -> Mux1/7
  FIRch24/1 -> Mux1/8
  Demux1/8 -> FIRch24/1
  Demux1/9 -> FIRch23/1
  FIRch23/1 -> Mux1/9
  FIRch22/1 -> Mux1/10
  Demux1/10 -> FIRch22/1
  Demux1/11 -> FIRch21/1
  FIRch21/1 -> Mux1/11
  FIRch20/1 -> Mux1/12
  Demux1/12 -> FIRch20/1
  FIRch19/1 -> Mux1/13
  Demux1/13 -> FIRch19/1
  FIRch18/1 -> Mux1/14
  Demux1/14 -> FIRch18/1
  Demux1/15 -> FIRch17/1
  FIRch17/1 -> Mux1/15
  Demux1/16 -> FIRch16/1
  Demux1/17 -> FIRch15/1
  Demux1/18 -> FIRch14/1
  Demux1/19 -> FIRch13/1
  Demux1/20 -> FIRch12/1
  Demux1/21 -> FIRch11/1
  Demux1/22 -> FIRch10/1
  Demux1/23 -> FIRch9/1
  Demux1/24 -> FIRch8/1
  Demux1/25 -> FIRch7/1
  Demux1/26 -> FIRch6/1
  Demux1/27 -> FIRch5/1
  Demux1/28 -> FIRch4/1
  Demux1/29 -> FIRch3/1
  Demux1/30 -> FIRch2/1
  Demux1/31 -> FIRch1/1
  Demux1/32 -> FIRch0/1
  FIRch16/1 -> Mux1/16
  FIRch15/1 -> Mux1/17
  FIRch14/1 -> Mux1/18
  FIRch13/1 -> Mux1/19
  FIRch12/1 -> Mux1/20
  FIRch11/1 -> Mux1/21
  FIRch10/1 -> Mux1/22
  FIRch9/1 -> Mux1/23
  FIRch8/1 -> Mux1/24
  FIRch7/1 -> Mux1/25
  FIRch6/1 -> Mux1/26
  FIRch5/1 -> Mux1/27
  FIRch4/1 -> Mux1/28
  FIRch3/1 -> Mux1/29
  FIRch2/1 -> Mux1/30
  FIRch1/1 -> Mux1/31
  FIRch0/1 -> Mux1/32
  Mux1/1 -> Flip1/1
  Flip1/1 -> IFFT1/1
  IFFT1/1 -> channelizer/1  "normal_channelizer"

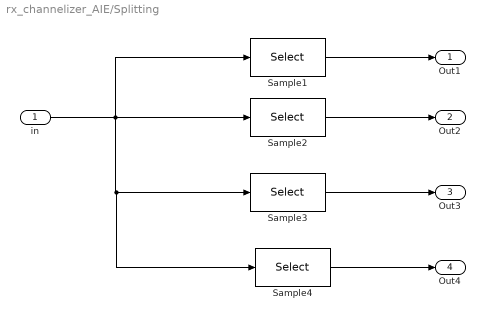
== system rx_channelizer_AIE/Splitting ==
  in : Inport
  Sample1 : Selector  InputPortWidth=1280  IndexOptions=Index vector (dialog)  Indices=1:4:1280  OutputSizes=1
  Sample2 : Selector  InputPortWidth=1280  IndexOptions=Index vector (dialog)  Indices=2:4:1280  OutputSizes=1
  Sample3 : Selector  InputPortWidth=1280  IndexOptions=Index vector (dialog)  Indices=3:4:1280  OutputSizes=1
  Sample4 : Selector  InputPortWidth=1280  IndexOptions=Index vector (dialog)  Indices=4:4:1280  OutputSizes=1
  Out1 : Outport
  Out2 : Outport  Port=2
  Out3 : Outport  Port=3
  Out4 : Outport  Port=4
  wires:
  in/1 -> Sample4/1, Sample3/1, Sample2/1, Sample1/1
  Sample2/1 -> Out2/1
  Sample1/1 -> Out1/1
  Sample3/1 -> Out3/1
  Sample4/1 -> Out4/1

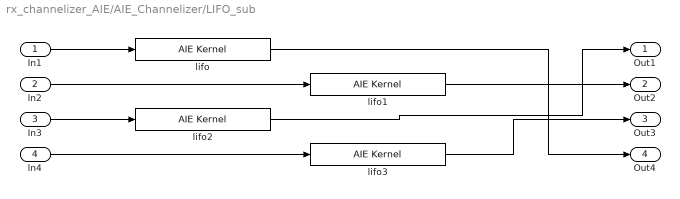
== system rx_channelizer_AIE/AIE_Channelizer/LIFO_sub ==
  In1 : Inport
  In2 : Inport  Port=2
  In3 : Inport  Port=3
  In4 : Inport  Port=4
  lifo : aieBasic/AIE Kernel  KernelAllAttrs=|  PortNames={'in'; 'out'}  PortSerializedTypes={'{R{Tadf::input_buffer{1{t{Scint32}}}}}'; '{R{Tadf::output_buffer{1{t{Scint32}}}}}'}  PortWindowSizes={3.200000000000000000e+02, 3.200000000000000000e+02}  PortWindowMargins={0.000000000000000000e+00, 0.000000000000000000e+00}  PortSynchronicities={'sync', 'sync'}  PortSignalSizes={0.000000000000000000e+00; 0.000000000000000000e+00}  FunctionTemplateSpecKind=implicit  FunctionTemplateParamNames={'FRAME_LENGTH'}  FunctionTemplateParamKinds={'nontype'}  FunctionTemplateParamTypes={'int'}  FunctionTemplateParamValues={'320'}  FunctionIndex=1  FunctionTabVisible=on  FunctionTemplateParamsVisible=on  FunctionDeclTypeOptions=|  FunctionDecl=|  FunctionTemplateParams={ 'FRAME_LENGTH', 'int', '320' }  FunctionTemplateParamsEnables={'off', 'off', 'on'}  PortAttrs={ 'input', 'in', 'adf::input_buffer< cint32 > &', '320', '0', 'sync', ''; 'output', 'out', 'adf::output_buffer< cint32 > &', '320', '', 'sync', '' }  PortAttrsEnables={'off', 'off', 'off', 'on', 'off', 'off', 'off';'off', 'off', 'off', 'on', 'off', 'off', 'off'}  SampleTime=-1  KernelHeaderFile=lifo.h  KernelFunction=lifo  KernelSourceFile=lifo.cc  KernelSearchPaths={}  PreProcOptions={}  blockJsonConstraints="{\"type\":\"constraint\",\"constraintType\":\"coreUtilization\",\"sid\":\"3263\",\"lhs\":{\"type\":\"runtimeRatio\",\"args\":{\"type\":\"kernel\",\"name\":\"rx_channelizer_AIE/AIEchannelizer/LIFO_sub/lifo\",\"sid\":\"3263\"}},\"rhs\":{\"type\":\"evaluable\",\"expr\":\"0.1\",\"value\":0.1},\"equality\":true}"
      KernelAllAttrs=|
      | s[12;12;9;9;19;14;21;23;21;23;24;21;15;17;12;24;26;26;26;27;28;9;21;23;23;23;24;25;14;19;19;29]@FunctionNameDeclFileNamePortNamesPortTypesPortSerializedTypesPortDirectionsPortWindowSizeEnablesPortWindowMarginEnablesPortBufferSizeEnablesPortBufferMarginEnablesPortSynchronicityEnablesPortSignalSizeEnablesPortBufferSizesPortBufferMarginsFunctionDeclFunctionTemplateSpecKindFunctionTemplateParamNamesFunctionTemplateParamKindsFunctionTemplateParamTypesFunctionTemplateParamValuesFunctionTemplateParamEnablesClassDeclClassTemplateSpecKindClassTemplateParamNamesClassTemplateParamKindsClassTemplateParamTypesClassTemplateParamValuesClassTemplateParamEnablesClassCtorDeclsClassCtorParamNamesClassCtorParamTypesClassCtorParamSerializedTypes[1 1]@C[32 1]@t4@lifot12@../../lifo.hC[2 1]@t2@int3@outC[2 1]@t29@adf::input_buffer< cint32 > &t30@adf::output_buffer< cint32 > &C[2 1]@t38@{R{Tadf::input_buffer{1{t{Scint32}}}}}t39@{R{Tadf::output_buffer{1{t{Scint32}}}}}C[2 1]@t5@inputt6@outputC[2 1]@l1@l1@C[2 1]@l1@l0@C[2 1]@l1@l1@C[2 1]@l0@l0@C[2 1]@l1@l1@C[2 1]@l0@l0@C[2 1]@nnC[2 1]@nnt110@template < int FRAME_LENGTH > 
      | void lifo(adf::input_buffer< cint32 > & in, adf::output_buffer< cint32 > & out)t8@implicitC[1 1]@t12@FRAME_LENGTHC[1 1]@t7@nontypeC[1 1]@t3@intC[1 1]@nC[1 1]@l1@nne[0 1]@e[0 1]@e[0 1]@e[0 1]@e[0 1]@e[0 1]@e[0 1]@e[0 1]@e[0 1]@
      FunctionDeclTypeOptions=|
      | C[1 1]@t112@template < int FRAME_LENGTH > 
      | void lifo(adf::input_buffer< cint32 > && in, adf::output_buffer< cint32 > && out)
      FunctionDecl=|
      | template < int FRAME_LENGTH > 
      | void lifo(adf::input_buffer< cint32 > && in, adf::output_buffer< cint32 > && out)
  lifo1 : aieBasic/AIE Kernel  KernelAllAttrs=|  PortNames={'in'; 'out'}  PortSerializedTypes={'{R{Tadf::input_buffer{1{t{Scint32}}}}}'; '{R{Tadf::output_buffer{1{t{Scint32}}}}}'}  PortWindowSizes={3.200000000000000000e+02, 3.200000000000000000e+02}  PortWindowMargins={0.000000000000000000e+00, 0.000000000000000000e+00}  PortSynchronicities={'sync', 'sync'}  PortSignalSizes={0.000000000000000000e+00; 0.000000000000000000e+00}  FunctionTemplateSpecKind=implicit  FunctionTemplateParamNames={'FRAME_LENGTH'}  FunctionTemplateParamKinds={'nontype'}  FunctionTemplateParamTypes={'int'}  FunctionTemplateParamValues={'320'}  FunctionIndex=1  FunctionTabVisible=on  FunctionTemplateParamsVisible=on  FunctionDeclTypeOptions=|  FunctionDecl=|  FunctionTemplateParams={ 'FRAME_LENGTH', 'int', '320' }  FunctionTemplateParamsEnables={'off', 'off', 'on'}  PortAttrs={ 'input', 'in', 'adf::input_buffer< cint32 > &', '320', '0', 'sync', ''; 'output', 'out', 'adf::output_buffer< cint32 > &', '320', '', 'sync', '' }  PortAttrsEnables={'off', 'off', 'off', 'on', 'off', 'off', 'off';'off', 'off', 'off', 'on', 'off', 'off', 'off'}  SampleTime=-1  KernelHeaderFile=lifo.h  KernelFunction=lifo  KernelSourceFile=lifo.cc  KernelSearchPaths={}  PreProcOptions={}  blockJsonConstraints="{\"type\":\"constraint\",\"constraintType\":\"coreUtilization\",\"sid\":\"3264\",\"lhs\":{\"type\":\"runtimeRatio\",\"args\":{\"type\":\"kernel\",\"name\":\"rx_channelizer_AIE/AIEchannelizer/LIFO_sub/lifo1\",\"sid\":\"3264\"}},\"rhs\":{\"type\":\"evaluable\",\"expr\":\"0.1\",\"value\":0.1},\"equality\":true}"
      KernelAllAttrs=|
      | s[12;12;9;9;19;14;21;23;21;23;24;21;15;17;12;24;26;26;26;27;28;9;21;23;23;23;24;25;14;19;19;29]@FunctionNameDeclFileNamePortNamesPortTypesPortSerializedTypesPortDirectionsPortWindowSizeEnablesPortWindowMarginEnablesPortBufferSizeEnablesPortBufferMarginEnablesPortSynchronicityEnablesPortSignalSizeEnablesPortBufferSizesPortBufferMarginsFunctionDeclFunctionTemplateSpecKindFunctionTemplateParamNamesFunctionTemplateParamKindsFunctionTemplateParamTypesFunctionTemplateParamValuesFunctionTemplateParamEnablesClassDeclClassTemplateSpecKindClassTemplateParamNamesClassTemplateParamKindsClassTemplateParamTypesClassTemplateParamValuesClassTemplateParamEnablesClassCtorDeclsClassCtorParamNamesClassCtorParamTypesClassCtorParamSerializedTypes[1 1]@C[32 1]@t4@lifot12@../../lifo.hC[2 1]@t2@int3@outC[2 1]@t29@adf::input_buffer< cint32 > &t30@adf::output_buffer< cint32 > &C[2 1]@t38@{R{Tadf::input_buffer{1{t{Scint32}}}}}t39@{R{Tadf::output_buffer{1{t{Scint32}}}}}C[2 1]@t5@inputt6@outputC[2 1]@l1@l1@C[2 1]@l1@l0@C[2 1]@l1@l1@C[2 1]@l0@l0@C[2 1]@l1@l1@C[2 1]@l0@l0@C[2 1]@nnC[2 1]@nnt110@template < int FRAME_LENGTH > 
      | void lifo(adf::input_buffer< cint32 > & in, adf::output_buffer< cint32 > & out)t8@implicitC[1 1]@t12@FRAME_LENGTHC[1 1]@t7@nontypeC[1 1]@t3@intC[1 1]@nC[1 1]@l1@nne[0 1]@e[0 1]@e[0 1]@e[0 1]@e[0 1]@e[0 1]@e[0 1]@e[0 1]@e[0 1]@
      FunctionDeclTypeOptions=|
      | C[1 1]@t112@template < int FRAME_LENGTH > 
      | void lifo(adf::input_buffer< cint32 > && in, adf::output_buffer< cint32 > && out)
      FunctionDecl=|
      | template < int FRAME_LENGTH > 
      | void lifo(adf::input_buffer< cint32 > && in, adf::output_buffer< cint32 > && out)
  lifo2 : aieBasic/AIE Kernel  KernelAllAttrs=|  PortNames={'in'; 'out'}  PortSerializedTypes={'{R{Tadf::input_buffer{1{t{Scint32}}}}}'; '{R{Tadf::output_buffer{1{t{Scint32}}}}}'}  PortWindowSizes={3.200000000000000000e+02, 3.200000000000000000e+02}  PortWindowMargins={0.000000000000000000e+00, 0.000000000000000000e+00}  PortSynchronicities={'sync', 'sync'}  PortSignalSizes={0.000000000000000000e+00; 0.000000000000000000e+00}  FunctionTemplateSpecKind=implicit  FunctionTemplateParamNames={'FRAME_LENGTH'}  FunctionTemplateParamKinds={'nontype'}  FunctionTemplateParamTypes={'int'}  FunctionTemplateParamValues={'320'}  FunctionIndex=1  FunctionTabVisible=on  FunctionTemplateParamsVisible=on  FunctionDeclTypeOptions=|  FunctionDecl=|  FunctionTemplateParams={ 'FRAME_LENGTH', 'int', '320' }  FunctionTemplateParamsEnables={'off', 'off', 'on'}  PortAttrs={ 'input', 'in', 'adf::input_buffer< cint32 > &', '320', '0', 'sync', ''; 'output', 'out', 'adf::output_buffer< cint32 > &', '320', '', 'sync', '' }  PortAttrsEnables={'off', 'off', 'off', 'on', 'off', 'off', 'off';'off', 'off', 'off', 'on', 'off', 'off', 'off'}  SampleTime=-1  KernelHeaderFile=lifo.h  KernelFunction=lifo  KernelSourceFile=lifo.cc  KernelSearchPaths={}  PreProcOptions={}  blockJsonConstraints="{\"type\":\"constraint\",\"constraintType\":\"coreUtilization\",\"sid\":\"3265\",\"lhs\":{\"type\":\"runtimeRatio\",\"args\":{\"type\":\"kernel\",\"name\":\"rx_channelizer_AIE/AIEchannelizer/LIFO_sub/lifo2\",\"sid\":\"3265\"}},\"rhs\":{\"type\":\"evaluable\",\"expr\":\"0.1\",\"value\":0.1},\"equality\":true}"
      KernelAllAttrs=|
      | s[12;12;9;9;19;14;21;23;21;23;24;21;15;17;12;24;26;26;26;27;28;9;21;23;23;23;24;25;14;19;19;29]@FunctionNameDeclFileNamePortNamesPortTypesPortSerializedTypesPortDirectionsPortWindowSizeEnablesPortWindowMarginEnablesPortBufferSizeEnablesPortBufferMarginEnablesPortSynchronicityEnablesPortSignalSizeEnablesPortBufferSizesPortBufferMarginsFunctionDeclFunctionTemplateSpecKindFunctionTemplateParamNamesFunctionTemplateParamKindsFunctionTemplateParamTypesFunctionTemplateParamValuesFunctionTemplateParamEnablesClassDeclClassTemplateSpecKindClassTemplateParamNamesClassTemplateParamKindsClassTemplateParamTypesClassTemplateParamValuesClassTemplateParamEnablesClassCtorDeclsClassCtorParamNamesClassCtorParamTypesClassCtorParamSerializedTypes[1 1]@C[32 1]@t4@lifot12@../../lifo.hC[2 1]@t2@int3@outC[2 1]@t29@adf::input_buffer< cint32 > &t30@adf::output_buffer< cint32 > &C[2 1]@t38@{R{Tadf::input_buffer{1{t{Scint32}}}}}t39@{R{Tadf::output_buffer{1{t{Scint32}}}}}C[2 1]@t5@inputt6@outputC[2 1]@l1@l1@C[2 1]@l1@l0@C[2 1]@l1@l1@C[2 1]@l0@l0@C[2 1]@l1@l1@C[2 1]@l0@l0@C[2 1]@nnC[2 1]@nnt110@template < int FRAME_LENGTH > 
      | void lifo(adf::input_buffer< cint32 > & in, adf::output_buffer< cint32 > & out)t8@implicitC[1 1]@t12@FRAME_LENGTHC[1 1]@t7@nontypeC[1 1]@t3@intC[1 1]@nC[1 1]@l1@nne[0 1]@e[0 1]@e[0 1]@e[0 1]@e[0 1]@e[0 1]@e[0 1]@e[0 1]@e[0 1]@
      FunctionDeclTypeOptions=|
      | C[1 1]@t112@template < int FRAME_LENGTH > 
      | void lifo(adf::input_buffer< cint32 > && in, adf::output_buffer< cint32 > && out)
      FunctionDecl=|
      | template < int FRAME_LENGTH > 
      | void lifo(adf::input_buffer< cint32 > && in, adf::output_buffer< cint32 > && out)
  lifo3 : aieBasic/AIE Kernel  KernelAllAttrs=|  PortNames={'in'; 'out'}  PortSerializedTypes={'{R{Tadf::input_buffer{1{t{Scint32}}}}}'; '{R{Tadf::output_buffer{1{t{Scint32}}}}}'}  PortWindowSizes={3.200000000000000000e+02, 3.200000000000000000e+02}  PortWindowMargins={0.000000000000000000e+00, 0.000000000000000000e+00}  PortSynchronicities={'sync', 'sync'}  PortSignalSizes={0.000000000000000000e+00; 0.000000000000000000e+00}  FunctionTemplateSpecKind=implicit  FunctionTemplateParamNames={'FRAME_LENGTH'}  FunctionTemplateParamKinds={'nontype'}  FunctionTemplateParamTypes={'int'}  FunctionTemplateParamValues={'320'}  FunctionIndex=1  FunctionTabVisible=on  FunctionTemplateParamsVisible=on  FunctionDeclTypeOptions=|  FunctionDecl=|  FunctionTemplateParams={ 'FRAME_LENGTH', 'int', '320' }  FunctionTemplateParamsEnables={'off', 'off', 'on'}  PortAttrs={ 'input', 'in', 'adf::input_buffer< cint32 > &', '320', '0', 'sync', ''; 'output', 'out', 'adf::output_buffer< cint32 > &', '320', '', 'sync', '' }  PortAttrsEnables={'off', 'off', 'off', 'on', 'off', 'off', 'off';'off', 'off', 'off', 'on', 'off', 'off', 'off'}  SampleTime=-1  KernelHeaderFile=lifo.h  KernelFunction=lifo  KernelSourceFile=lifo.cc  KernelSearchPaths={}  PreProcOptions={}  blockJsonConstraints="{\"type\":\"constraint\",\"constraintType\":\"coreUtilization\",\"sid\":\"3266\",\"lhs\":{\"type\":\"runtimeRatio\",\"args\":{\"type\":\"kernel\",\"name\":\"rx_channelizer_AIE/AIEchannelizer/LIFO_sub/lifo3\",\"sid\":\"3266\"}},\"rhs\":{\"type\":\"evaluable\",\"expr\":\"0.1\",\"value\":0.1},\"equality\":true}"
      KernelAllAttrs=|
      | s[12;12;9;9;19;14;21;23;21;23;24;21;15;17;12;24;26;26;26;27;28;9;21;23;23;23;24;25;14;19;19;29]@FunctionNameDeclFileNamePortNamesPortTypesPortSerializedTypesPortDirectionsPortWindowSizeEnablesPortWindowMarginEnablesPortBufferSizeEnablesPortBufferMarginEnablesPortSynchronicityEnablesPortSignalSizeEnablesPortBufferSizesPortBufferMarginsFunctionDeclFunctionTemplateSpecKindFunctionTemplateParamNamesFunctionTemplateParamKindsFunctionTemplateParamTypesFunctionTemplateParamValuesFunctionTemplateParamEnablesClassDeclClassTemplateSpecKindClassTemplateParamNamesClassTemplateParamKindsClassTemplateParamTypesClassTemplateParamValuesClassTemplateParamEnablesClassCtorDeclsClassCtorParamNamesClassCtorParamTypesClassCtorParamSerializedTypes[1 1]@C[32 1]@t4@lifot12@../../lifo.hC[2 1]@t2@int3@outC[2 1]@t29@adf::input_buffer< cint32 > &t30@adf::output_buffer< cint32 > &C[2 1]@t38@{R{Tadf::input_buffer{1{t{Scint32}}}}}t39@{R{Tadf::output_buffer{1{t{Scint32}}}}}C[2 1]@t5@inputt6@outputC[2 1]@l1@l1@C[2 1]@l1@l0@C[2 1]@l1@l1@C[2 1]@l0@l0@C[2 1]@l1@l1@C[2 1]@l0@l0@C[2 1]@nnC[2 1]@nnt110@template < int FRAME_LENGTH > 
      | void lifo(adf::input_buffer< cint32 > & in, adf::output_buffer< cint32 > & out)t8@implicitC[1 1]@t12@FRAME_LENGTHC[1 1]@t7@nontypeC[1 1]@t3@intC[1 1]@nC[1 1]@l1@nne[0 1]@e[0 1]@e[0 1]@e[0 1]@e[0 1]@e[0 1]@e[0 1]@e[0 1]@e[0 1]@
      FunctionDeclTypeOptions=|
      | C[1 1]@t112@template < int FRAME_LENGTH > 
      | void lifo(adf::input_buffer< cint32 > && in, adf::output_buffer< cint32 > && out)
      FunctionDecl=|
      | template < int FRAME_LENGTH > 
      | void lifo(adf::input_buffer< cint32 > && in, adf::output_buffer< cint32 > && out)
  Out1 : Outport
  Out2 : Outport  Port=2
  Out3 : Outport  Port=3
  Out4 : Outport  Port=4
  wires:
  In2/1 -> lifo1/1
  lifo1/1 -> Out2/1
  In4/1 -> lifo3/1
  In1/1 -> lifo/1
  lifo3/1 -> Out3/1
  lifo/1 -> Out4/1
  In3/1 -> lifo2/1
  lifo2/1 -> Out1/1
